simulink model "smooth_pursuit"  (R2018b)
settings: Solver=ode45  StartTime=0.0  StopTime=10  RelTol=1e-3  EnableMultiTasking=on
values from neighbouring files (symbols this model uses):
  deta1 = 0.16    [smoothparamter.m]
  deta2 = 0.08    [smoothparamter.m]
  k1 = 0.55    [smoothparamter.m]
  k2 = 1    [smoothparamter.m]
  kd = 0    [smoothparamter.m]
  kp = 0.45    [smoothparamter.m]
  te = 0.015    [smoothparamter.m]
  tn = 0.07    [smoothparamter.m]
libraries: simulink x1
settings Model: Creator=Zigzag-pc  LastModifiedBy=Jorish
settings DataIOCC: LimitDataPoints=on  SaveFormat=Array  InspectSignalLogs=on
settings OptimizationCC: LifeSpan=inf
settings DebuggingCC: SolverPrmCheckMsg=warning  SFUnexpectedBacktrackingDiag=warning  SFNoUnconditionalDefaultTransitionDiag=warning
settings HardwareCC: ProdBitPerPointer=32  ProdBitPerSizeT=32  ProdBitPerPtrDiffT=32  ProdLargestAtomicFloat=None  ProdIntDivRoundTo=Undefined  ProdEndianess=Unspecified  ProdWordSize=32  ProdHWDeviceType=32-bit Generic
settings ModelReferenceCC: PropagateSignalLabelsOutOfModel=off
settings SFSimCC: SimUseLocalCustomCode=off
settings RTWCC: RTWUseLocalCustomCode=off
settings CodeAppCC: StateflowObjectComments=on
settings GRTTargetCC: TargetLangStandard=C89/C90 (ANSI)  GeneratePreprocessorConditionals=Disable all
settings ConfigComp: CovMetricSettings=dw  CovHtmlReporting=on  CovSaveCumulativeToWorkspaceVar=on  CovSaveSingleToWorkspaceVar=on  CovExternalEMLEnable=off  CovSFcnEnable=off

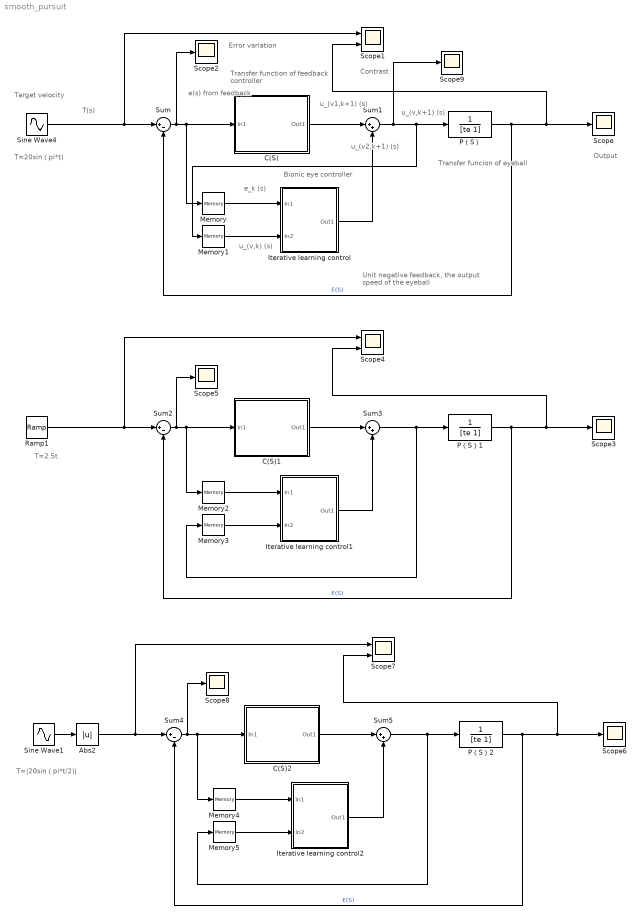
== system smooth_pursuit ==
  note: Transfer function
      | of feedback controller
  note: Unit negative feedback,
      | the output speed of the eyeball
  note: Bionic eye controller
  note: Transfer funcion
      | of eyeball
  note: Target velocity
  note: e_k (s)
  note: u_(v1,k+1) (s)
  note: T=2.5t
  note: T=20sin（pi*t)
  note: Error
      | variation
  note: Output
  note: Contrast
  note: e(s) from
      | feedback
  note: T(s)
  note: T=|20sin（pi*t/2)|
  note: u_(v,k+1) (s)
  note: u_(v2,k+1) (s)
  note: u_(v,k) (s)
  Abs2 : Abs
  C(S) : Subsystem
  C(S)1 : Subsystem
  C(S)2 : Subsystem
  Iterative learning control : Subsystem
  Iterative learning control1 : Subsystem
  Iterative learning control2 : Subsystem
  Memory : Memory  InitialCondition=1.5  InheritSampleTime=on
  Memory1 : Memory  InitialCondition=25  InheritSampleTime=on
  Memory2 : Memory  InitialCondition=1  InheritSampleTime=on
  Memory3 : Memory  InitialCondition=25  InheritSampleTime=on
  Memory4 : Memory  InitialCondition=10  InheritSampleTime=on
  Memory5 : Memory  InitialCondition=50  InheritSampleTime=on
  P（S） : TransferFcn  Denominator=[te 1]
  P（S）1 : TransferFcn  Denominator=[te 1]
  P（S）2 : TransferFcn  Denominator=[te 1]
  Ramp1 : simulink/Sources/Ramp  slope=2.5  start=0  InitialOutput=0
  Scope{,2..3,5..6,8..9} (7 alike) : Scope
  Scope1 : Scope  NumInputPorts=2
  Scope4 : Scope  NumInputPorts=2
  Scope7 : Scope  NumInputPorts=2
  Sine Wave1 : Sin  Amplitude=20  Frequency=pi/2  SampleTime=0
  Sine Wave4 : Sin  Amplitude=20  Frequency=pi  SampleTime=0
  Sum : Sum  Inputs=|+-
  Sum1 : Sum  Inputs=|++
  Sum2 : Sum  Inputs=|+-
  Sum3 : Sum  Inputs=|++
  Sum4 : Sum  Inputs=|+-
  Sum5 : Sum  Inputs=|++
  wires:
  Sum/1 -> Scope2/1, Memory/1, C(S)/1(In1)
  C(S)/1(Out1) -> Sum1/1
  Sum1/1 -> Scope9/1, P（S）/1, Memory1/1
  P（S）/1 -> Scope1/2, Scope/1, Sum/2  "E(S)"
  Memory/1 -> Iterative learning control/1(In1)
  Memory1/1 -> Iterative learning control/2(In2)
  Iterative learning control/1(Out1) -> Sum1/2
  Sine Wave4/1 -> Scope1/1, Sum/1
  Sum2/1 -> Scope5/1, Memory2/1, C(S)1/1(In1)
  C(S)1/1(Out1) -> Sum3/1
  P（S）1/1 -> Scope4/2, Scope3/1, Sum2/2  "E(S)"
  Memory2/1 -> Iterative learning control1/1(In1)
  Memory3/1 -> Iterative learning control1/2(In2)
  Iterative learning control1/1(Out1) -> Sum3/2
  Ramp1/1 -> Scope4/1, Sum2/1
  Sum4/1 -> Scope8/1, Memory4/1, C(S)2/1(In1)
  C(S)2/1(Out1) -> Sum5/1
  Sum5/1 -> P（S）2/1, Memory5/1
  P（S）2/1 -> Scope7/2, Scope6/1, Sum4/2  "E(S)"
  Memory4/1 -> Iterative learning control2/1(In1)
  Memory5/1 -> Iterative learning control2/2(In2)
  Iterative learning control2/1(Out1) -> Sum5/2
  Abs2/1 -> Scope7/1, Sum4/1
  Sine Wave1/1 -> Abs2/1
  Sum3/1 -> P（S）1/1, Memory3/1

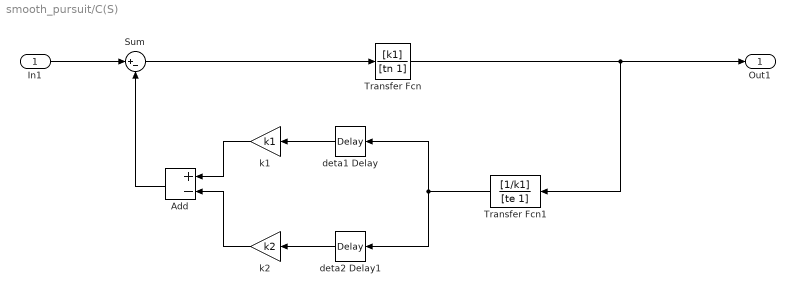
== system smooth_pursuit/C(S) ==
  In1 : Inport
  Add : Sum  Inputs=+-
  Sum : Sum  Inputs=|+-
  Transfer Fcn : TransferFcn  Numerator=[k1]  Denominator=[tn 1]
  Transfer Fcn1 : TransferFcn  Numerator=[1/k1]  Denominator=[te 1]
  deta1 Delay : TransportDelay  DelayTime=deta1
  deta2 Delay1 : TransportDelay  DelayTime=deta2
  k1 : Gain  Gain=k1
  k2 : Gain  Gain=k2
  Out1 : Outport
  wires:
  deta1 Delay/1 -> k1/1
  k1/1 -> Add/1
  k2/1 -> Add/2
  Transfer Fcn/1 -> Out1/1, Transfer Fcn1/1
  deta2 Delay1/1 -> k2/1
  Transfer Fcn1/1 -> deta2 Delay1/1, deta1 Delay/1
  Add/1 -> Sum/2
  Sum/1 -> Transfer Fcn/1
  In1/1 -> Sum/1

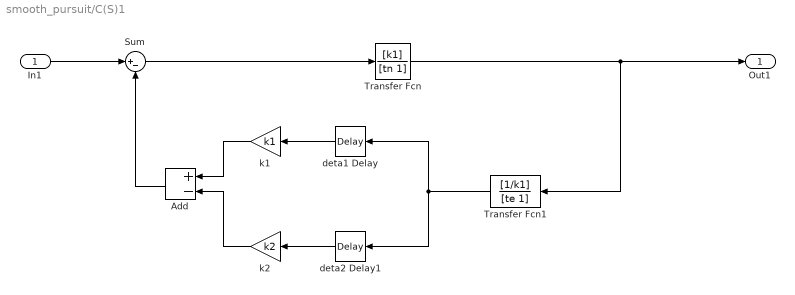
== system smooth_pursuit/C(S)1 ==
  In1 : Inport
  Add : Sum  Inputs=+-
  Sum : Sum  Inputs=|+-
  Transfer Fcn : TransferFcn  Numerator=[k1]  Denominator=[tn 1]
  Transfer Fcn1 : TransferFcn  Numerator=[1/k1]  Denominator=[te 1]
  deta1 Delay : TransportDelay  DelayTime=deta1
  deta2 Delay1 : TransportDelay  DelayTime=deta2
  k1 : Gain  Gain=k1
  k2 : Gain  Gain=k2
  Out1 : Outport
  wires:
  deta1 Delay/1 -> k1/1
  k1/1 -> Add/1
  k2/1 -> Add/2
  Transfer Fcn/1 -> Out1/1, Transfer Fcn1/1
  deta2 Delay1/1 -> k2/1
  Transfer Fcn1/1 -> deta2 Delay1/1, deta1 Delay/1
  Add/1 -> Sum/2
  Sum/1 -> Transfer Fcn/1
  In1/1 -> Sum/1

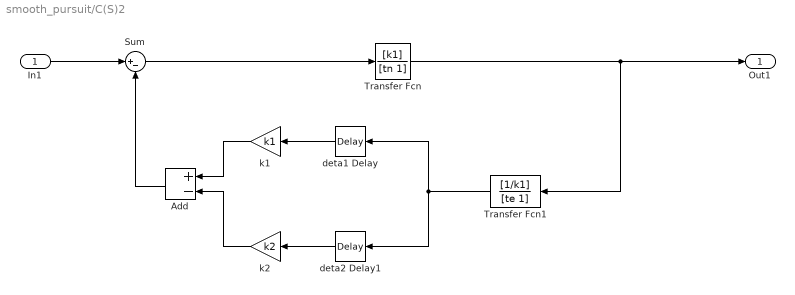
== system smooth_pursuit/C(S)2 ==
  In1 : Inport
  Add : Sum  Inputs=+-
  Sum : Sum  Inputs=|+-
  Transfer Fcn : TransferFcn  Numerator=[k1]  Denominator=[tn 1]
  Transfer Fcn1 : TransferFcn  Numerator=[1/k1]  Denominator=[te 1]
  deta1 Delay : TransportDelay  DelayTime=deta1
  deta2 Delay1 : TransportDelay  DelayTime=deta2
  k1 : Gain  Gain=k1
  k2 : Gain  Gain=k2
  Out1 : Outport
  wires:
  deta1 Delay/1 -> k1/1
  k1/1 -> Add/1
  k2/1 -> Add/2
  Transfer Fcn/1 -> Out1/1, Transfer Fcn1/1
  deta2 Delay1/1 -> k2/1
  Transfer Fcn1/1 -> deta2 Delay1/1, deta1 Delay/1
  Add/1 -> Sum/2
  Sum/1 -> Transfer Fcn/1
  In1/1 -> Sum/1

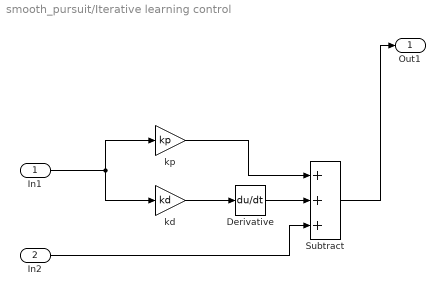
== system smooth_pursuit/Iterative learning control ==
  In1 : Inport
  In2 : Inport  Port=2
  Derivative : Derivative  CoefficientInTFapproximation=-1
  Subtract : Sum  Inputs=+++
  kd : Gain  Gain=kd
  kp : Gain  Gain=kp
  Out1 : Outport
  wires:
  In1/1 -> kp/1, kd/1
  Subtract/1 -> Out1/1
  kd/1 -> Derivative/1
  kp/1 -> Subtract/1
  Derivative/1 -> Subtract/2
  In2/1 -> Subtract/3

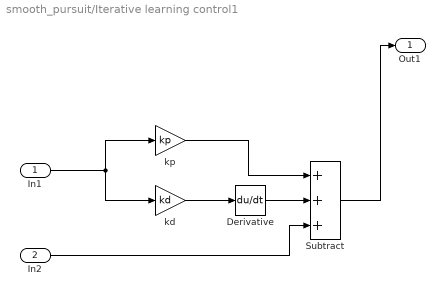
== system smooth_pursuit/Iterative learning control1 ==
  In1 : Inport
  In2 : Inport  Port=2
  Derivative : Derivative  CoefficientInTFapproximation=-1
  Subtract : Sum  Inputs=+++
  kd : Gain  Gain=kd
  kp : Gain  Gain=kp
  Out1 : Outport
  wires:
  In1/1 -> kp/1, kd/1
  Subtract/1 -> Out1/1
  kd/1 -> Derivative/1
  kp/1 -> Subtract/1
  Derivative/1 -> Subtract/2
  In2/1 -> Subtract/3

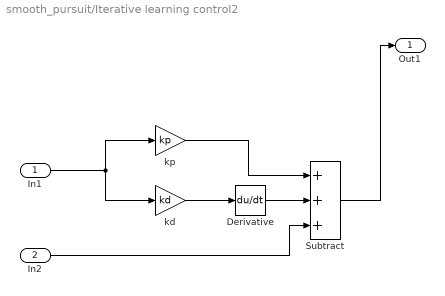
== system smooth_pursuit/Iterative learning control2 ==
  In1 : Inport
  In2 : Inport  Port=2
  Derivative : Derivative  CoefficientInTFapproximation=-1
  Subtract : Sum  Inputs=+++
  kd : Gain  Gain=kd
  kp : Gain  Gain=kp
  Out1 : Outport
  wires:
  In1/1 -> kp/1, kd/1
  Subtract/1 -> Out1/1
  kd/1 -> Derivative/1
  kp/1 -> Subtract/1
  Derivative/1 -> Subtract/2
  In2/1 -> Subtract/3
